simulink model "TestForce3Axis"  (R2022b)
settings: Solver=FixedStepAuto  StartTime=0.0  StopTime=50  FixedStep=simulator.TimeStep  RelTol=1e-3  EnableMultiTasking=on
undefined symbols (not defined in the file): simulator
settings Model: SimulationMode=external  Creator=At  LastModifiedBy=ateay
settings SolverCC: AlgebraicLoopSolver=TrustRegion
settings DataIOCC: SaveFormat=StructureWithTime  ReturnWorkspaceOutputs=off
settings OptimizationCC: BlockReduction=off  OptimizeBlockIOStorage=off  BufferReuse=off  GlobalBufferReuse=off  ExpressionFolding=off  LocalBlockOutputs=off
settings DebuggingCC: UnconnectedInputMsg=warning  UnconnectedOutputMsg=warning  UnconnectedLineMsg=warning  SFMachineParentedDataDiag=warning  ArithmeticOperatorsInVariantConditions=warning
settings HardwareCC: ProdBitPerPointer=32  ProdBitPerSizeT=32  ProdBitPerPtrDiffT=32  ProdLargestAtomicFloat=None  ProdWordSize=32  ProdLongLongMode=on  ProdHWDeviceType=Generic->32-bit x86 compatible
settings ModelReferenceCC: EnableRefExpFcnMdlSchedulingChecks=on  ModelReferenceNumInstancesAllowed=Single
settings SFSimCC: SimUseLocalCustomCode=off  CustomCodeUndefinedFunction=UseInterfaceOnly
settings RTWCC: Description=Simulink Real-Time  SystemTargetFile=slrt.tlc  TemplateMakefile=slrt_default_tmf  RTWUseLocalCustomCode=off  RTWCompilerOptimization=on
settings CodeAppCC: StateflowObjectComments=on
settings SimulinkRealTimeCC: OptimizeReductions=off  RL32LogBufSizeModifier=1000000

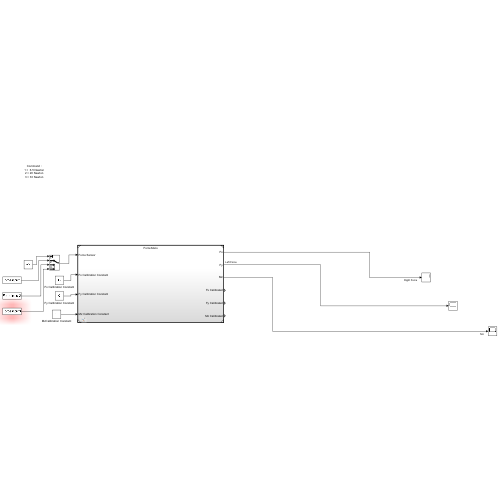
[thumbnail: Simulink's stored preview of the top-level diagram]
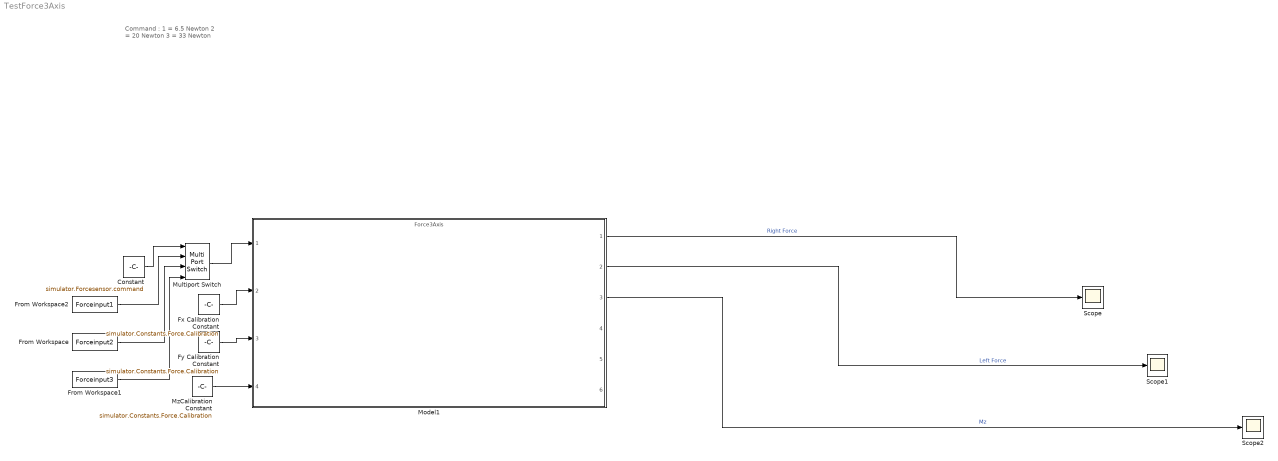
== system TestForce3Axis ==
  note: Command :
      | 1 =  6.5 Newton
      | 2 = 20 Newton
      | 3 = 33 Newton
  Constant : Constant  Value=simulator.Forcesensor.command
  From Workspace : FromWorkspace  VariableName=Forceinput2
  From Workspace1 : FromWorkspace  VariableName=Forceinput3
  From Workspace2 : FromWorkspace  VariableName=Forceinput1
  Fx Calibration Constant : Constant  Value=simulator.Constants.Force.Calibration  mask{Parameter1=0}
      mask DialogControl CalibrationConstant Prompt: Calibration Constant
  Fy Calibration Constant : Constant  Value=simulator.Constants.Force.Calibration  mask{Parameter1=0}
      mask DialogControl CalibrationConstant Prompt: Calibration Constant
  Model1 : ModelReference  ModelNameDialog=Force3Axis.slx  SimulationMode=Normal  ModelReferenceVersion=12.2
  Multiport Switch : MultiPortSwitch  SaturateOnIntegerOverflow=off  InputSameDT=off
  MzCalibration Constant : Constant  Value=simulator.Constants.Force.Calibration  mask{Parameter1=0}
      mask DialogControl CalibrationConstant Prompt: Calibration Constant
  Scope : Scope
  Scope1 : Scope
  Scope2 : Scope
  wires:
  Model1/1 -> Scope/1  "Right Force"
  Model1/3 -> Scope2/1  "Mz"
  Model1/2 -> Scope1/1  "Left Force"
  From Workspace2/1 -> Multiport Switch/2
  Constant/1 -> Multiport Switch/1
  From Workspace/1 -> Multiport Switch/3
  From Workspace1/1 -> Multiport Switch/4
  Multiport Switch/1 -> Model1/1
  Fx Calibration Constant/1 -> Model1/2
  Fy Calibration Constant/1 -> Model1/3
  MzCalibration Constant/1 -> Model1/4
